simulink model "Smart_City_QCar1_self_driving_stack"  (R2024b)
settings: Solver=ode1  StartTime=0.0  StopTime=inf  FixedStep=Controller_Sample_Time  RelTol=1e-3  EnableMultiTasking=on
values from neighbouring files (symbols this model uses):
  angles_qcar1 = angles_new_qcar1(2: length (angles_new_qcar1), width (angles_new_qcar1)-5)    [Setup_QCar1and2_params.m]
  Audio_Sample_Time = 0.3    [Setup_QCar1and2_params.m]
  cal_pos = [0, 0, 0]    [Setup_QCar1and2_params.m]
  cameraStepSize = 3e-2    (= 0.03)    [Setup_QCar1and2_params.m]
  Cobra_Start = [0 0 0 0 0 0 0 0 0 0 0 0 ... (192000 elements, 192000x1)]    [QCar_Sounds.mat]
  Controller_Sample_Time = CSI_Sample_Time/10    (= 0.00166666666667)    [Setup_QCar1and2_params.m]
  CSI_Sample_Time = 1/60    (= 0.0166666666667)    [Setup_QCar1and2_params.m]
  GyroKF_P0 = eye(2)    [Setup_QCar1and2_params.m]
  GyroKF_Q = diag([0.01, 0.001])    [Setup_QCar1and2_params.m]
  GyroKF_R = 0.01    [Setup_QCar1and2_params.m]
  GyroKF_X0 = [0;0]    [Setup_QCar1and2_params.m]
  honk = [0.01708984375 0.0179443359375 0.018798828125 0.019775390625 0.0209655761719 0.0218505859375 0.0221557617188 0.0223693847656 0.022705078125 0.023681640625 0.0252075195312 0.0257263183594 ... (43568 elements, 21784x2)]    [QCar_Sounds.mat]
  ImageDisplay_Sample_Time = CSI_Sample_Time*6    (= 0.1)    [Setup_QCar1and2_params.m]
  Initialization_Time = 5    [Setup_QCar1and2_params.m]
  LiDAR_Sample_Time = CSI_Sample_Time*3    (= 0.05)    [Setup_QCar1and2_params.m]
  map_mask = [1 1 1 0 0 1 0]    [Setup_QCar1and2_params.m]
  NN_Sample_Time = RealSense_Sample_Time*1    (= 0.0333333333333)    [Setup_QCar1and2_params.m]
  path_x = [0.826 0.836 0.846 0.856 0.866 0.876 0.886 0.896 0.906 0.916 0.926 0.936 ... (740 elements, 740x1)]    [SDCS_Paths_7.mat]
  path_x2 = [-0.614 -0.604 -0.594 -0.584 -0.574 -0.564 -0.554 -0.544 -0.534 -0.524 -0.514 -0.504 ... (1090 elements, 1090x1)]    [SDCS_Paths_7.mat]
  path_x3 = [-0.614 -0.603821428571 -0.593642857143 -0.583464285714 -0.573285714286 -0.563107142857 -0.552928571429 -0.54275 -0.532571428571 -0.522392857143 -0.512214285714 -0.502035714286 ... (714 elements, 714x1)]    [SDCS_Paths_7.mat]
  path_x4 = [-0.614 -0.604 -0.594 -0.584 -0.574 -0.564 -0.554 -0.544 -0.534 -0.524 -0.514 -0.504 ... (1761 elements, 1761x1)]    [SDCS_Paths_7.mat]
  path_x5 = [1.436 1.42588571429 1.41577142857 1.40565714286 1.39554285714 1.38542857143 1.37531428571 1.3652 1.35508571429 1.34497142857 1.33485714286 1.32474285714 ... (574 elements, 574x1)]    [SDCS_Paths_7.mat]
  path_x6 = [1.436 1.42588571429 1.41577142857 1.40565714286 1.39554285714 1.38542857143 1.37531428571 1.3652 1.35508571429 1.34497142857 1.33485714286 1.32474285714 ... (1288 elements, 1288x1)]    [SDCS_Paths_7.mat]
  path_x7 = [-1.5778487585 -1.56959877056 -1.56127865467 -1.55288878259 -1.54442952915 -1.53590127231 -1.52730439309 -1.51863927561 -1.50990630701 -1.50110587746 -1.49223838016 -1.4833042113 ... (2260 elements, 2260x1)]    [SDCS_Paths_7.mat]
  path_y = [-1.0887 -1.0887 -1.0887 -1.0887 -1.0887 -1.0887 -1.0887 -1.0887 -1.0887 -1.0887 -1.0887 -1.0887 ... (740 elements, 740x1)]    [SDCS_Paths_7.mat]
  path_y2 = [-1.0887 -1.0887 -1.0887 -1.0887 -1.0887 -1.0887 -1.0887 -1.0887 -1.0887 -1.0887 -1.0887 -1.0887 ... (1090 elements, 1090x1)]    [SDCS_Paths_7.mat]
  path_y3 = [-1.0887 -1.0887 -1.0887 -1.0887 -1.0887 -1.0887 -1.0887 -1.0887 -1.0887 -1.0887 -1.0887 -1.0887 ... (714 elements, 714x1)]    [SDCS_Paths_7.mat]
  path_y4 = [-1.0887 -1.0887 -1.0887 -1.0887 -1.0887 -1.0887 -1.0887 -1.0887 -1.0887 -1.0887 -1.0887 -1.0887 ... (1761 elements, 1761x1)]    [SDCS_Paths_7.mat]
  path_y5 = [-0.8157 -0.8157 -0.8157 -0.8157 -0.8157 -0.8157 -0.8157 -0.8157 -0.8157 -0.8157 -0.8157 -0.8157 ... (574 elements, 574x1)]    [SDCS_Paths_7.mat]
  path_y6 = [-0.8157 -0.8157 -0.8157 -0.8157 -0.8157 -0.8157 -0.8157 -0.8157 -0.8157 -0.8157 -0.8157 -0.8157 ... (1288 elements, 1288x1)]    [SDCS_Paths_7.mat]
  path_y7 = [-0.614490295955 -0.61974988896 -0.624981792226 -0.630185771997 -0.635361595765 -0.640509032279 -0.645627851559 -0.6507178249 -0.655778724888 -0.660810325409 -0.665812401655 -0.670784730139 ... (2260 elements, 2260x1)]    [SDCS_Paths_7.mat]
  put_me_down = [0 0 0 0 0 0 0 0 0 0 0 0 ... (335870 elements, 167935x2)]    [QCar_Sounds.mat]
  qcar1_lidar_to_map_rotation = pi/2    (= 1.57079632679)    [Setup_QCar1and2_params.m]
  QCarEKF_L = 0.24    [Setup_QCar1and2_params.m]
  QCarEKF_P0 = eye(3)    [Setup_QCar1and2_params.m]
  QCarEKF_Q = diag([0.00001, 0.00001, 0.00001])    [Setup_QCar1and2_params.m]
  QCarEKF_R_combined = diag([0.1, 0.1, 0.01])    [Setup_QCar1and2_params.m]
  QCarEKF_R_heading = diag(0.1)    [Setup_QCar1and2_params.m]
  QcarKF_X0 = [0; 0; 0]    [Setup_QCar1and2_params.m]
  range_qcar1 = distance_new_qcar1(2: length (distance_new_qcar1), width (distance_new_qcar1)-5)    [Setup_QCar1and2_params.m]
  RealSense_Sample_Time = CSI_Sample_Time*2    (= 0.0333333333333)    [Setup_QCar1and2_params.m]
undefined symbols (not defined in the file or in its folder): DiscIntNeverNeededParam, gcbh, HIL, Joystick_Sample_Time, JPEG, Point, qc_get_step_size, video_display_show
libraries: quarc_library x63, simulink_extras x12, simulink x8
(part 1 of 5)
settings Model: SimulationMode=external  ExtModeTrigDuration=10000  Creator=PKaram  LastModifiedBy=user
settings SolverCC: AlgebraicLoopSolver=TrustRegion  PositivePriorityOrder=on  AutoInsertRateTranBlk=on
settings DataIOCC: ReturnWorkspaceOutputs=off
settings DebuggingCC: ParameterPrecisionLossMsg=none  UnconnectedInputMsg=warning  UnconnectedOutputMsg=warning  UnconnectedLineMsg=warning  ArithmeticOperatorsInVariantConditions=warning
settings HardwareCC: ProdBitPerLong=64  ProdLargestAtomicFloat=None  ProdEndianess=Unspecified  ProdHWDeviceType=Generic->64-bit Embedded Processor (LP64)
settings ModelReferenceCC: EnableRefExpFcnMdlSchedulingChecks=on
settings SFSimCC: SimUseLocalCustomCode=off  CustomCodeUndefinedFunction=UseInterfaceOnly
settings RTWCC: Description=QUARC Linux Nvidia Target (QCar) Using Toolchain  SystemTargetFile=quarc_linux_nvidia.tlc  TemplateMakefile=quarc_linux_nvidia_tmf  RTWUseLocalCustomCode=off  Toolchain=QUARC linux_nvidia | gmake (64-bit Windows)  BuildConfiguration=Faster Runs  GPUComputeCapability=3.5
settings CodeAppCC: StateflowObjectComments=on
settings STFCustomTargetCC: TargetLangStandard=C99 (ISO)  ConcurrentExecutionCompliant=on  GRTInterface=on  UseToolchainInfoCompliant=on  SystemTargetFile=quarc_linux_nvidia.tlc
settings GRTTargetCC: ParMdlRefBuildCompliant=off  CompOptLevelCompliant=off  CombineOutputUpdateFcns=off  MatFileLogging=off  CPPClassGenCompliant=off  GRTInterface=on  ExtMode=on  ExtModeMexFile=quarc_comm  ExtModeMexArgs='-w -d /tmp -uri %u', 'tcpip://192.168.2.12:17001'
settings ConfigComp: CovMetricSettings=dswe

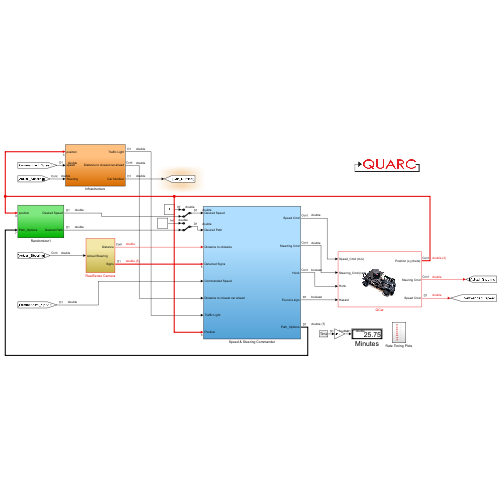
[thumbnail: Simulink's stored preview of the top-level diagram]
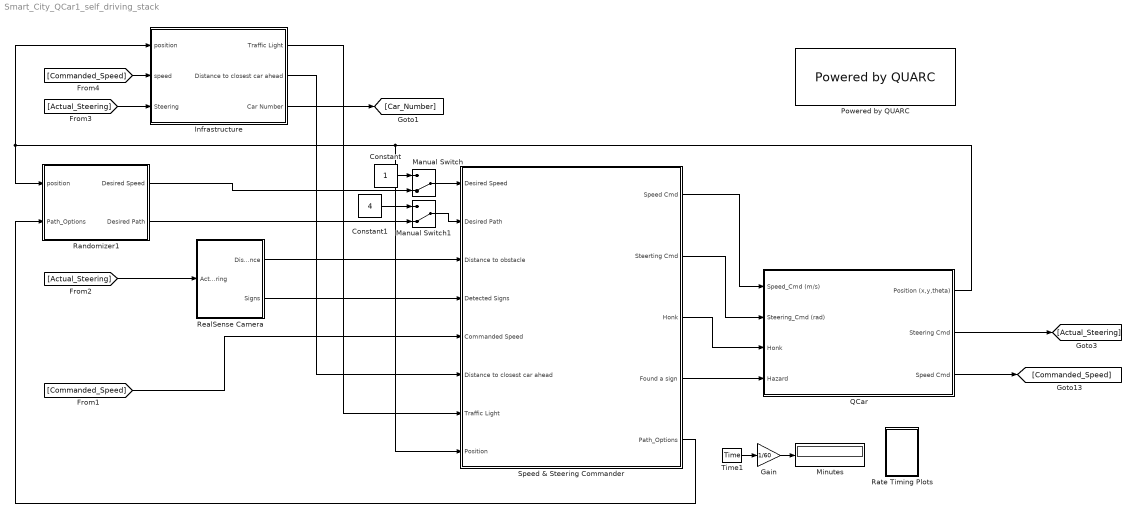
== system Smart_City_QCar1_self_driving_stack ==
  Constant : Constant
  Constant1 : Constant  Value=4
  Gain : Gain  Gain=1/60
  Infrastructure : Subsystem
  Manual Switch : ManualSwitch  CurrentSetting=0
  Manual Switch1 : ManualSwitch  CurrentSetting=0
  Minutes : Display
  Powered by QUARC : quarc_library/Logos/Powered by QUARC
  QCar : Subsystem
      mask Display: image('QCar.png'); % Use "Edit Image" on toolstrip to change.
  Randomizer1 : Subsystem
  Rate Timing Plots : Subsystem
  RealSense Camera : Subsystem
  Speed & Steering Commander : Subsystem
  Time1 : quarc_library/Sources/Time/Time  time_source=Wall clock  sample_time=qc_get_step_size
  wires:
  QCar/2(Steering Cmd) -> [Actual_Steering]
  QCar/3(Speed Cmd) -> [Commanded_Speed]
  Time1/1 -> Gain/1
  Gain/1 -> Minutes/1
  Infrastructure/1(Traffic Light) -> Speed & Steering Commander/7(Traffic Light)
  Infrastructure/2(Distance to closest car ahead) -> Speed & Steering Commander/6(Distance to closest car ahead)
  Infrastructure/3(Car Number) -> [Car_Number]
  [Actual_Steering] -> RealSense Camera/1(Actual Steering)
  [Commanded_Speed] -> Infrastructure/2("speed ")
  QCar/1(Position (x,y,theta)) -> Speed & Steering Commander/8(Position), Randomizer1/1(position), Infrastructure/1(position)
  [Actual_Steering] -> Infrastructure/3(Steering)
  [Commanded_Speed] -> Speed & Steering Commander/5(Commanded Speed)
  RealSense Camera/2(Signs) -> Speed & Steering Commander/4(Detected Signs)
  RealSense Camera/1(Distance) -> Speed & Steering Commander/3(Distance to obstacle)
  Speed & Steering Commander/4(Found a sign) -> QCar/4(Hazard)
  Speed & Steering Commander/1(Speed Cmd) -> QCar/1(Speed_Cmd (m/s))
  Speed & Steering Commander/2(Steerting Cmd) -> QCar/2(Steering_Cmd (rad))
  Speed & Steering Commander/3(Honk) -> QCar/3(Honk)
  Speed & Steering Commander/5(Path_Options) -> Randomizer1/2(Path_Options)
  Manual Switch/1 -> Speed & Steering Commander/1(Desired Speed)
  Randomizer1/1(Desired Speed) -> Manual Switch/2
  Constant/1 -> Manual Switch/1
  Randomizer1/2(Desired Path) -> Manual Switch1/2
  Constant1/1 -> Manual Switch1/1
  Manual Switch1/1 -> Speed & Steering Commander/2(Desired Path)

== system Smart_City_QCar1_self_driving_stack/Infrastructure ==
  note: Send Position and Heading to Ground Station
  note: Find:
      | 1 - Traffic light states (bool)
      | 2 - Distance to closes car for adaptive cruise control
      | 3 - Car number
  note: Get Data
  note: Make sure to change the port for each car:
      | 1: 1111
      | 2: 2222
      | 3: 3333
      | 4: 4444
      | 5: 5555
  position : Inport
  "speed " : Inport  Port=2
  Steering : Inport  Port=3
  Add : Sum
  Constant1 : Constant  Value=10
  Constant2 : Constant
  Constant4 : Constant
  Constant6 : Constant  Value=10
  Constant7 : Constant
  Demux : Demux  Outputs=[10 1 1]
  Display : Display
  Display1 : Display
  Display2 : Display
      settings: Decimation=100
  Find Closest Car : Subsystem
  Gain1 : Gain  Gain=.11537*1
  Mux : Mux  Inputs=2
  Mux3 : Mux  Inputs=2
  Saturation : Saturate  UpperLimit=1  LowerLimit=0
  Saturation1 : Saturate  UpperLimit=5  LowerLimit=1
  Second-Order Low-Pass Filter : quarc_library/Continuous/Second-Order Low-Pass Filter  params_source=External (input ports)  input_width=1  input_zeta=1  input_init=0
  Second-Order Low-Pass Filter1 : quarc_library/Continuous/Second-Order Low-Pass Filter  params_source=External (input ports)  input_width=1  input_zeta=1  input_init=0
  Selector : Selector  InputPortWidth=3  IndexOptions=Index vector (dialog)  Indices=1:2  OutputSizes=1
  Selector1 : Selector  InputPortWidth=3  IndexOptions=Index vector (dialog)  Indices=3  OutputSizes=1
  Stream Server : quarc_library/Communications/Basic/Stream Server  uri_source=Specify via dialog (do not evaluate)  uri=tcpip://remotehost:1111?nagle='off'  send_buffer_size=1460  receive_buffer_size=1460  byte_order=little endian (Intel - LSB first)  optimization=Minimum latency  send_options=Send most recent data  receive_options=Receive most recent data  default_value=10* ones (1,12)  sample_time=qc_get_step_size  active=off  implementation=Use blocking I/O in a separate thread  send_fifo_size=1  receive_fifo_size=1  send_priority=0  receive_priority=0  send_dimensions=off  receive_dimensions=off  max_dimensions=-1  data_type=Inherited via back propagation  type_expr=BusObject
      settings: AttributesFormatString="\"tcpip://remotehost:1111?nagle='off'\""
  Sum1 : Sum  Inputs=+-
  Trigonometric Function : Trigonometry  Operator=cos
  Trigonometric Function1 : Trigonometry
  Traffic Light : Outport
  Distance to closest car ahead : Outport  Port=2
  Car Number : Outport  Port=3
  wires:
  Constant7/1 -> Second-Order Low-Pass Filter/3
  Constant4/1 -> Stream Server/2
  Stream Server/1 -> Display2/1
  Constant6/1 -> Second-Order Low-Pass Filter/2
  position/1 -> Selector1/1, Selector/1
  Selector/1 -> [xy]
  Selector1/1 -> [mod_heading]
  Second-Order Low-Pass Filter/1 -> Display/1, Distance to closest car ahead/1
  Constant1/1 -> Second-Order Low-Pass Filter1/2
  "speed "/1 -> Second-Order Low-Pass Filter1/1, Second-Order Low-Pass Filter1/4
  Stream Server/4 -> Demux/1, Display1/1
  [xy] -> Find Closest Car/2(car_position)
  Constant2/1 -> Second-Order Low-Pass Filter1/3
  Second-Order Low-Pass Filter1/1 -> Find Closest Car/1("speed ")
  Find Closest Car/1(distance) -> Second-Order Low-Pass Filter/1, Second-Order Low-Pass Filter/4
  Add/1 -> Find Closest Car/3(car_heading)
  [mod_heading] -> Add/1
  Steering/1 -> Add/2
  Demux/1 -> Find Closest Car/4(other_car_position)
  Demux/2 -> Saturation/1
  Saturation/1 -> Traffic Light/1
  Mux/1 -> Stream Server/1
  Sum1/1 -> Mux/1
  [mod_heading] -> Mux/2
  Demux/3 -> Saturation1/1
  Saturation1/1 -> Car Number/1, Find Closest Car/5(car_index)
  [mod_heading] -> Trigonometric Function1/1, Trigonometric Function/1
  Mux3/1 -> Gain1/1
  Trigonometric Function1/1 -> Mux3/2
  [xy] -> Sum1/1
  Gain1/1 -> Sum1/2
  Trigonometric Function/1 -> Mux3/1

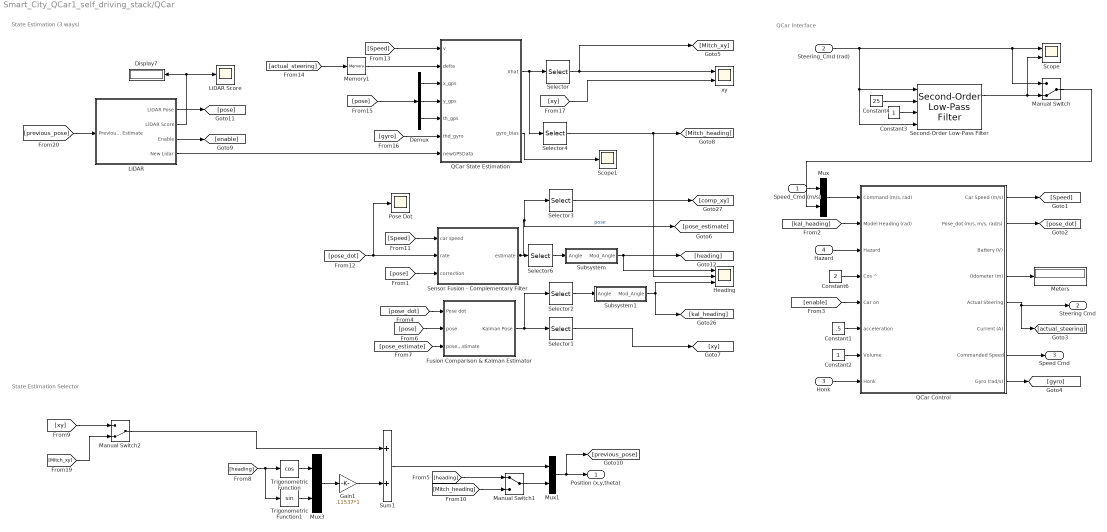
== system Smart_City_QCar1_self_driving_stack/QCar ==
  note: QCar Interface
  note: State Estimation (3 ways)
  note: State Estimation Selector
  Speed_Cmd (m/s) : Inport
  Steering_Cmd (rad) : Inport  Port=2
  Honk : Inport  Port=3
  Hazard : Inport  Port=4
  Constant1 : Constant  Value=.5
  Constant2 : Constant
  Constant3 : Constant
  Constant4 : Constant  Value=25
  Constant6 : Constant  Value=2
  Demux : Demux  Outputs=3
  Display7 : Display
  Fusion Comparison & Kalman Estimator : Subsystem
  Gain1 : Gain  Gain=.11537*1
  Heading : Scope  NumInputPorts=3
  LiDAR : Subsystem
  LiDAR Score : Scope
  Manual Switch : ManualSwitch  CurrentSetting=0
  Manual Switch1 : ManualSwitch
  Manual Switch2 : ManualSwitch  CurrentSetting=0
  Memory1 : Memory
  Meters : Display
  Mux : Mux  Inputs=2
  Mux1 : Mux  Inputs=2
  Mux3 : Mux  Inputs=2
  Pose Dot : Scope
  QCar Control : Subsystem
  QCar State Estimation : Subsystem
  Scope : Scope  NumInputPorts=2
  Scope1 : Scope
  Second-Order Low-Pass Filter : quarc_library/Continuous/Second-Order Low-Pass Filter  params_source=External (input ports)  input_width=1  input_zeta=1  input_init=0
  Selector : Selector  InputPortWidth=3  IndexOptions=Index vector (dialog)  Indices=1:2  OutputSizes=1
  Selector1 : Selector  InputPortWidth=3  IndexOptions=Index vector (dialog)  Indices=1:2  OutputSizes=1
  Selector2 : Selector  InputPortWidth=3  IndexOptions=Index vector (dialog)  Indices=3  OutputSizes=1
  Selector3 : Selector  InputPortWidth=3  IndexOptions=Index vector (dialog)  Indices=1:2  OutputSizes=1
  Selector4 : Selector  InputPortWidth=3  IndexOptions=Index vector (dialog)  Indices=3  OutputSizes=1
  Selector6 : Selector  InputPortWidth=3  IndexOptions=Index vector (dialog)  Indices=3  OutputSizes=1
  Sensor Fusion - Complementary Filter : Subsystem
  Subsystem : Subsystem
  Subsystem1 : Subsystem
  Sum1 : Sum
  Trigonometric Function : Trigonometry  Operator=cos
  Trigonometric Function1 : Trigonometry
  "xy " : Scope  NumInputPorts=2
  Position (x,y,theta) : Outport
  Steering Cmd : Outport  Port=2
  Speed Cmd : Outport  Port=3
  wires:
  Mux/1 -> QCar Control/1("Command (m/s, rad)")
  Speed_Cmd (m/s)/1 -> Mux/1
  LiDAR/2("LiDAR Score ") -> LiDAR Score/1, Display7/1
  LiDAR/1(LiDAR Pose) -> [pose]
  LiDAR/3(Enable) -> [enable]
  [pose] -> Fusion Comparison & Kalman Estimator/2(pose)
  Selector3/1 -> [comp_xy]
  [Speed] -> Sensor Fusion - Complementary Filter/1(car speed)
  Sensor Fusion - Complementary Filter/1(estimate) -> Selector3/1, [pose_estimate], Selector6/1  "pose"
  [pose_dot] -> Pose Dot/1, Sensor Fusion - Complementary Filter/2(rate)
  Selector6/1 -> Subsystem/1(Angle)
  Fusion Comparison & Kalman Estimator/1(Kalman Pose) -> Selector2/1, Selector1/1
  [pose] -> Sensor Fusion - Complementary Filter/3(correction)
  Subsystem/1(Mod_Angle) -> Heading/1, [heading]
  [pose_estimate] -> Fusion Comparison & Kalman Estimator/3(pose estimate)
  Selector2/1 -> Subsystem1/1(Angle)
  [pose_dot] -> Fusion Comparison & Kalman Estimator/1(Pose dot)
  QCar Control/1(Car Speed (m/s)) -> [Speed]
  QCar Control/2("Pose_dot (m/s, m/s, rad/s)") -> [pose_dot]
  QCar Control/5(Actual Steering) -> [actual_steering], Steering Cmd/1
  QCar Control/7(Commanded Speed) -> Speed Cmd/1
  Selector1/1 -> [xy]
  [kal_heading] -> QCar Control/2(Model Heading (rad))
  Subsystem1/1(Mod_Angle) -> Heading/3, [kal_heading]
  Constant6/1 -> QCar Control/4(Cos ^)
  Constant1/1 -> QCar Control/6(acceleration)
  [enable] -> QCar Control/5(Car on)
  Constant2/1 -> QCar Control/7(Volume)
  Honk/1 -> QCar Control/8(Honk)
  Mux1/1 -> [previous_pose], Position (x,y,theta)/1
  QCar Control/4(Odometer (m)) -> Meters/1
  Hazard/1 -> QCar Control/3(Hazard)
  Gain1/1 -> Sum1/2
  Trigonometric Function/1 -> Mux3/1
  Mux3/1 -> Gain1/1
  Trigonometric Function1/1 -> Mux3/2
  [heading] -> Trigonometric Function1/1, Trigonometric Function/1
  Sum1/1 -> Mux1/1
  Manual Switch/1 -> Mux/2
  Second-Order Low-Pass Filter/1 -> Scope/2, Manual Switch/2
  Steering_Cmd (rad)/1 -> Manual Switch/1, Scope/1, Second-Order Low-Pass Filter/1, Second-Order Low-Pass Filter/4
  Constant3/1 -> Second-Order Low-Pass Filter/3
  Constant4/1 -> Second-Order Low-Pass Filter/2
  Manual Switch1/1 -> Mux1/2
  [heading] -> Manual Switch1/1
  [Mitch_heading] -> Manual Switch1/2
  [Speed] -> QCar State Estimation/1(v)
  Demux/1 -> QCar State Estimation/3(x_gps)
  Demux/2 -> QCar State Estimation/4(y_gps)
  Demux/3 -> QCar State Estimation/5(th_gps)
  [pose] -> Demux/1
  QCar Control/8(Gyro (rad/s)) -> [gyro]
  [gyro] -> QCar State Estimation/6(thd_gyro)
  LiDAR/4(New Lidar) -> QCar State Estimation/7(newGPSData)
  QCar State Estimation/1(Xhat) -> Selector4/1, Selector/1
  [xy] -> "xy "/2
  Selector4/1 -> Heading/2, [Mitch_heading]
  QCar State Estimation/2(gyro_bias) -> Scope1/1
  Selector/1 -> [Mitch_xy], "xy "/1
  Manual Switch2/1 -> Sum1/1
  [xy] -> Manual Switch2/1
  [Mitch_xy] -> Manual Switch2/2
  [actual_steering] -> Memory1/1
  Memory1/1 -> QCar State Estimation/2(delta)
  [previous_pose] -> LiDAR/1(Previous Estimate)

== system Smart_City_QCar1_self_driving_stack/Randomizer1 ==
  note: Tunable Params
  position : Inport
  Path_Options : Inport  Port=2
  Base Speed : Constant  Value=.35
  Compare To Constant : simulink/Logic and Bit Operations/Compare To Constant  relop=<  const=0  OutDataTypeStr=boolean
  Compare To Constant1 : simulink/Logic and Bit Operations/Compare To Constant  relop=>  const=-0.75  OutDataTypeStr=boolean
  Compare To Constant2 : simulink/Logic and Bit Operations/Compare To Constant  relop=<  const=-0.9  OutDataTypeStr=boolean
  Display : Display
  Display1 : Display
  Logical Operator : Logic  AllPortsSameDT=off  OutDataTypeStr=boolean
  Logical Operator1 : Logic  AllPortsSameDT=off  OutDataTypeStr=boolean
  MATLAB Function : MATLAB Function  TreatAsAtomicUnit=on
  Memory1 : Memory  InitialCondition=2  InheritSampleTime=on  LinearizeMemory=on  LinearizeAsDelay=on
  Memory2 : Memory  InitialCondition=1  InheritSampleTime=on  LinearizeMemory=on  LinearizeAsDelay=on
  Subsystem1 : Subsystem
  Terminator : Terminator
  Time b/w Path Changes : Constant  Value=3
  X : Selector  InputPortWidth=3  IndexOptions=Index vector (dialog)  Indices=[1]  OutputSizes=1
  Y : Selector  InputPortWidth=3  IndexOptions=Index vector (dialog)  Indices=[2]  OutputSizes=1
  multiply : Product  Inputs=**
  select which which path set to use : Subsystem  TreatAsAtomicUnit=on
  Desired Speed : Outport
  Desired Path : Outport  Port=2
  wires:
  Memory1/1 -> MATLAB Function/1(Previous_Path)
  Memory2/1 -> MATLAB Function/2(Previous_Speed)
  Time b/w Path Changes/1 -> Subsystem1/1(Random Period)
  Subsystem1/1(RisingEdgeTrigger) -> MATLAB Function/5(randomize)
  Base Speed/1 -> MATLAB Function/4(Speed_Cmd_Base)
  MATLAB Function/2(Desired_Speed) -> Desired Speed/1, Memory2/1, Display1/1
  MATLAB Function/1(Desired_Path) -> Memory1/1, Desired Path/1, Display/1
  MATLAB Function/3(Accel_Limit) -> Terminator/1
  X/1 -> Compare To Constant1/1, Compare To Constant/1
  Logical Operator/1 -> Logical Operator1/1
  Compare To Constant1/1 -> Logical Operator/2
  position/1 -> X/1, Y/1
  Logical Operator1/1 -> select which which path set to use/Trigger
  select which which path set to use/1(map mask) -> multiply/1
  Y/1 -> Compare To Constant2/1
  Compare To Constant/1 -> Logical Operator/1
  Compare To Constant2/1 -> Logical Operator1/2
  Path_Options/1 -> multiply/2
  multiply/1 -> MATLAB Function/3(Path_Options)

== system Smart_City_QCar1_self_driving_stack/Rate Timing Plots ==
  Audio : Scope
  CSI : Scope
  Control : Scope
  Image Displays : Scope
  Joystick : Scope  Commented=on
  LCD : Scope
  LiDAR : Scope
  NN Rate : Scope
  RealSense : Scope
  monitorTiming : Subsystem
  monitorTiming1 : Subsystem
  monitorTiming2 : Subsystem
  monitorTiming3 : Subsystem
  monitorTiming4 : Subsystem  Commented=on
  monitorTiming5 : Subsystem
  monitorTiming6 : Subsystem
  monitorTiming7 : Subsystem
  monitorTiming8 : Subsystem
  wires:
  monitorTiming/1(Timing (s)) -> CSI/1
  monitorTiming1/1(Timing (s)) -> Control/1
  monitorTiming3/1(Timing (s)) -> Image Displays/1
  monitorTiming4/1(Timing (s)) -> Joystick/1
  monitorTiming2/1(Timing (s)) -> RealSense/1
  monitorTiming5/1(Timing (s)) -> LiDAR/1
  monitorTiming6/1(Timing (s)) -> NN Rate/1
  monitorTiming7/1(Timing (s)) -> LCD/1
  monitorTiming8/1(Timing (s)) -> Audio/1

== system Smart_City_QCar1_self_driving_stack/RealSense Camera ==
  note: Capture Realsense and get object distance
  Actual Steering : Inport
  Constant8 : Constant  Value=50
  Constant9 : Constant
  NN Classification : Scope
  Newer Depth : Subsystem  LoadFcn=set_param(gcbh, 'UserData', gcb);  StartFcn=video_display_show([gcb, '/Video Display'], 'add', gcb);  mask(Video Compressed Display){algorithm=JPEG, quality=50, sample_time=-1, use_hardware=on}
      mask prompts: algorithm "Compression algorithm:"; quality "Compression quality (0-100):"; sample_time "Sample time (seconds):"; use_hardware "Use hardware acceleration for video display"
      mask help: Displays a video stream on the host, using compression to minimize bandwidth.
      mask init:
      | qc_set_display('Video\nCompressed\nDisplay');
      settings: UndoDeleteFcn=set_param(gcbh, 'UserData', gcb);  OpenFcn=video_display_show([gcb, '/Video Display'], 'show', gcb);  PreDeleteFcn=video_display_show([gcb, '/Video Display'], 'delete');
      settings: CopyFcn=|
      | set_param(gcbh, 'UserData', gcb);
      | set_param(gcbh, 'LinkStatus', 'none');
      settings: NameChangeFcn=|
      | video_display_show([get_param(gcbh, 'UserData'), '/Video Display'], 'rename', [gcb, '/Video Display']);
      | video_display_show([gcb, '/Video Display'], 'add', gcb);
      | set_param(gcbh, 'UserData', gcb);
      mask Help: web(qc_get_block_help_path(gcb));
      mask TypeOptions algorithm: Image Compress/algorithm
      mask TypeOptions quality: Image Compress/quality
      mask TypeOptions sample_time: Video Display/sample_time
      mask TypeOptions use_hardware: Video Display/use_hardware
      mask Display:
      | patch([0.98591 0.98591 0.62618 0.59072 0.56147   0.536   0.536  0.5441 0.56912 0.59207 0.60881 0.62276 0.63527 0.64364  0.6485  0.6485 0.64706 0.64499 0.63662 0.62411 0.61232 0.59837 0.58307 0.56147   0.536   0.536  0.5441  0.5747 0.60953 0.63662 0.67001  0.7034 0.72851 0.75425 0.77927 0.80294 0.82454 0.84119 0.85865 0.87395 0.88574 0.89339  0.8969 0.89969 0.89969 0.89267  0.8816 0.87044 0.85649  0.8384 0.81824 0.80294 0.78764 0.77513 0.76676 0.75776 0.76397 0.77513 0.79178 0.80987 0.82796 0.84326 0.86207 0.98528],[0.18689 0.05522 0.05522 0.05171 0.05171    0.05 0.18338 0.18338 0.19148 0.20435 0.22298 0.24863 0.28589 0.33125 0.38138 0.55139 0.59801 0.63761 0.68189 0.72149 0.74939 0.76694 0.77855 0.79367 0.79952 0.92768 0.92768 0.92768 0.92417 0.92066 0.91364  0.9032 0.89384 0.88106 0.86594 0.85073 0.82634 0.80537 0.77855 0.74363 0.70403 0.65858 0.61079 0.59099 0.41513 0.37202 0.31847 0.29048 0.25556 0.23342  0.2102 0.19382 0.18221 0.17285 0.16943 0.16124  0.1589 0.16241 0.16709 0.17168  0.1787 0.18221 0.18689 0.18689],[0.9,0.90,0.91])
      | patch([0.536 0.52601 0.46823 0.44528 0.41603 0.39101 0.35555 0.33116 0.31451 0.29291  0.2804 0.26717 0.25322 0.23999 0.22406 0.20732 0.19337 0.17528 0.15935 0.14396 0.13217 0.11759 0.10922 0.10085 0.09671 0.09392 0.09041 0.08906 0.08906 0.09464  0.0995 0.10778 0.11894 0.13145 0.14675 0.16349 0.17672 0.19409 0.20732 0.22406 0.23999 0.26159 0.27833 0.29849 0.31793 0.33602 0.35411 0.37085 0.39245 0.41603   0.536   0.536 0.53159 0.46409   0.446 0.42026 0.39587 0.37571 0.36113 0.34925 0.34088 0.33809 0.33809 0.34088 0.34583 0.35627 0.36392 0.38129 0.39587 0.41117 0.42719 0.44672  0.4676 0.48353 0.48353 0.52394   0.536],[0.05 0.04829 0.04712 0.04712 0.04829 0.05063 0.05405 0.05873 0.06107 0.06692 0.07043 0.07619 0.08087 0.08672 0.09482 0.10652 0.11696 0.13325  0.1508 0.17168 0.19499 0.22415 0.25439 0.28472 0.31379 0.35456 0.38489 0.41513 0.58055 0.63878 0.68774 0.72149 0.75641 0.78089 0.80537 0.82859 0.84029 0.85658 0.86594 0.87404  0.8834 0.89267 0.90086 0.90788 0.91247 0.91832 0.92066   0.923 0.92651 0.92768 0.92768 0.79952 0.79952 0.79952 0.79718 0.78899 0.77153 0.75056 0.72149 0.68072 0.62249  0.5549 0.41396 0.37085 0.33242 0.28121 0.25205 0.22181 0.20552 0.19499 0.18572 0.18221 0.17753 0.17636 0.17753  0.1787  0.1787],[0.9,0.90,0.91])
      | disp('Video\nCompressed\nDisplay');
  RGB : Subsystem  LoadFcn=set_param(gcbh, 'UserData', gcb);  StartFcn=video_display_show([gcb, '/Video Display'], 'add', gcb);  mask(Video Compressed Display){algorithm=JPEG, quality=50, sample_time=-1, use_hardware=on}
      mask prompts: algorithm "Compression algorithm:"; quality "Compression quality (0-100):"; sample_time "Sample time (seconds):"; use_hardware "Use hardware acceleration for video display"
      mask help: Displays a video stream on the host, using compression to minimize bandwidth.
      mask init:
      | qc_set_display('Video\nCompressed\nDisplay');
      settings: UndoDeleteFcn=set_param(gcbh, 'UserData', gcb);  OpenFcn=video_display_show([gcb, '/Video Display'], 'show', gcb);  PreDeleteFcn=video_display_show([gcb, '/Video Display'], 'delete');
      settings: CopyFcn=|
      | set_param(gcbh, 'UserData', gcb);
      | set_param(gcbh, 'LinkStatus', 'none');
      settings: NameChangeFcn=|
      | video_display_show([get_param(gcbh, 'UserData'), '/Video Display'], 'rename', [gcb, '/Video Display']);
      | video_display_show([gcb, '/Video Display'], 'add', gcb);
      | set_param(gcbh, 'UserData', gcb);
      mask Help: web(qc_get_block_help_path(gcb));
      mask TypeOptions algorithm: Image Compress/algorithm
      mask TypeOptions quality: Image Compress/quality
      mask TypeOptions sample_time: Video Display/sample_time
      mask TypeOptions use_hardware: Video Display/use_hardware
      mask Display:
      | patch([0.98591 0.98591 0.62618 0.59072 0.56147   0.536   0.536  0.5441 0.56912 0.59207 0.60881 0.62276 0.63527 0.64364  0.6485  0.6485 0.64706 0.64499 0.63662 0.62411 0.61232 0.59837 0.58307 0.56147   0.536   0.536  0.5441  0.5747 0.60953 0.63662 0.67001  0.7034 0.72851 0.75425 0.77927 0.80294 0.82454 0.84119 0.85865 0.87395 0.88574 0.89339  0.8969 0.89969 0.89969 0.89267  0.8816 0.87044 0.85649  0.8384 0.81824 0.80294 0.78764 0.77513 0.76676 0.75776 0.76397 0.77513 0.79178 0.80987 0.82796 0.84326 0.86207 0.98528],[0.18689 0.05522 0.05522 0.05171 0.05171    0.05 0.18338 0.18338 0.19148 0.20435 0.22298 0.24863 0.28589 0.33125 0.38138 0.55139 0.59801 0.63761 0.68189 0.72149 0.74939 0.76694 0.77855 0.79367 0.79952 0.92768 0.92768 0.92768 0.92417 0.92066 0.91364  0.9032 0.89384 0.88106 0.86594 0.85073 0.82634 0.80537 0.77855 0.74363 0.70403 0.65858 0.61079 0.59099 0.41513 0.37202 0.31847 0.29048 0.25556 0.23342  0.2102 0.19382 0.18221 0.17285 0.16943 0.16124  0.1589 0.16241 0.16709 0.17168  0.1787 0.18221 0.18689 0.18689],[0.9,0.90,0.91])
      | patch([0.536 0.52601 0.46823 0.44528 0.41603 0.39101 0.35555 0.33116 0.31451 0.29291  0.2804 0.26717 0.25322 0.23999 0.22406 0.20732 0.19337 0.17528 0.15935 0.14396 0.13217 0.11759 0.10922 0.10085 0.09671 0.09392 0.09041 0.08906 0.08906 0.09464  0.0995 0.10778 0.11894 0.13145 0.14675 0.16349 0.17672 0.19409 0.20732 0.22406 0.23999 0.26159 0.27833 0.29849 0.31793 0.33602 0.35411 0.37085 0.39245 0.41603   0.536   0.536 0.53159 0.46409   0.446 0.42026 0.39587 0.37571 0.36113 0.34925 0.34088 0.33809 0.33809 0.34088 0.34583 0.35627 0.36392 0.38129 0.39587 0.41117 0.42719 0.44672  0.4676 0.48353 0.48353 0.52394   0.536],[0.05 0.04829 0.04712 0.04712 0.04829 0.05063 0.05405 0.05873 0.06107 0.06692 0.07043 0.07619 0.08087 0.08672 0.09482 0.10652 0.11696 0.13325  0.1508 0.17168 0.19499 0.22415 0.25439 0.28472 0.31379 0.35456 0.38489 0.41513 0.58055 0.63878 0.68774 0.72149 0.75641 0.78089 0.80537 0.82859 0.84029 0.85658 0.86594 0.87404  0.8834 0.89267 0.90086 0.90788 0.91247 0.91832 0.92066   0.923 0.92651 0.92768 0.92768 0.79952 0.79952 0.79952 0.79718 0.78899 0.77153 0.75056 0.72149 0.68072 0.62249  0.5549 0.41396 0.37085 0.33242 0.28121 0.25205 0.22181 0.20552 0.19499 0.18572 0.18221 0.17753 0.17636 0.17753  0.1787  0.1787],[0.9,0.90,0.91])
      | disp('Video\nCompressed\nDisplay');
  Rate Transition : RateTransition
  Rate Transition2 : RateTransition
  Rate Transition4 : RateTransition
  RealSense Capture : Subsystem
  Second-Order Low-Pass Filter2 : quarc_library/Continuous/Second-Order Low-Pass Filter  params_source=External (input ports)  input_width=1  input_zeta=1  input_init=0
  Terminator : Terminator
  Transfer Fcn : TransferFcn  Numerator=[10]  Denominator=[1 10]
  obstacleDetection Markham March 22 : Subsystem
  to 16Hz4 : RateTransition  OutPortSampleTime=ImageDisplay_Sample_Time
  Distance : Outport
  Signs : Outport  Port=2
  wires:
  Transfer Fcn/1 -> Rate Transition4/1
  Actual Steering/1 -> Transfer Fcn/1
  Constant9/1 -> Second-Order Low-Pass Filter2/3
  obstacleDetection Markham March 22/2(distance (m)) -> Rate Transition2/1
  Rate Transition2/1 -> Second-Order Low-Pass Filter2/4, Second-Order Low-Pass Filter2/1
  to 16Hz4/1 -> Newer Depth/1(In1)
  obstacleDetection Markham March 22/1(imageDepthForDisplay) -> to 16Hz4/1
  Second-Order Low-Pass Filter2/2 -> Terminator/1
  RealSense Capture/1(New) -> obstacleDetection Markham March 22/Enable
  RealSense Capture/2(Depth) -> obstacleDetection Markham March 22/1(imageDepth)
  Rate Transition4/1 -> obstacleDetection Markham March 22/2(steering (rad))
  Constant8/1 -> Second-Order Low-Pass Filter2/2
  Second-Order Low-Pass Filter2/1 -> Distance/1
  RealSense Capture/3(RGB Image) -> RGB/1(In1)
  RealSense Capture/4(Sign Probabilities) -> Rate Transition/1, NN Classification/1
  Rate Transition/1 -> Signs/1

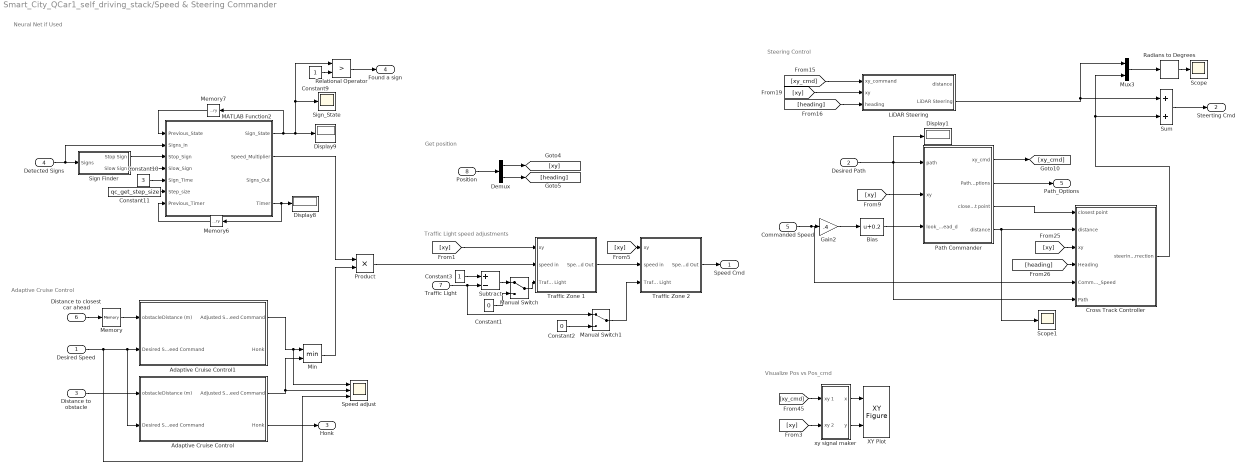
== system Smart_City_QCar1_self_driving_stack/Speed & Steering Commander ==
  note: Get position
  note: Steering Control
  note: Visualize Pos vs Pos_cmd
  note: Traffic Light speed adjustments
  note: Adaptive Cruise Control
  note: Neural Net if Used
  Desired Speed : Inport
  Desired Path : Inport  Port=2
  Distance to obstacle : Inport  Port=3
  Detected Signs : Inport  Port=4
  Commanded Speed : Inport  Port=5
  Distance to closest car ahead : Inport  Port=6
  Traffic Light : Inport  Port=7
  Position : Inport  Port=8
  Adaptive Cruise Control : Subsystem
  Adaptive Cruise Control1 : Subsystem
  Bias : Bias  Bias=0.2  SaturateOnIntegerOverflow=off
  Constant1 : Constant  Value=0
  Constant10 : Constant  Value=3
  Constant11 : Constant  Value=qc_get_step_size
  Constant2 : Constant  Value=0
  Constant3 : Constant
  Constant9 : Constant
  Cross Track Controller : Subsystem
  Demux : Demux  Outputs=2
  Display1 : Display
  Display8 : Display
  Display9 : Display
  Gain2 : Gain  Gain=.4
  LiDAR Steering : Subsystem
  MATLAB Function2 : MATLAB Function  TreatAsAtomicUnit=on
  Manual Switch : ManualSwitch
  Manual Switch1 : ManualSwitch
  Memory : Memory  InheritSampleTime=on  LinearizeMemory=on  LinearizeAsDelay=on
  Memory6 : Memory  InheritSampleTime=on  LinearizeMemory=on  LinearizeAsDelay=on
  Memory7 : Memory  InitialCondition=1  InheritSampleTime=on  LinearizeMemory=on  LinearizeAsDelay=on
  Min : MinMax  Inputs=2
  Mux3 : Mux  Inputs=2
  Path Commander : Subsystem
  Product : Product
  Radians to Degrees : simulink_extras/Transformations/Radians to Degrees
  Relational Operator : RelationalOperator  Operator=>  OutDataTypeStr=boolean  RndMeth=Simplest  InputSameDT=off
  Scope : Scope
  Scope1 : Scope
  Sign Finder : Subsystem
  Sign_State : Scope
  Speed adjust : Scope  NumInputPorts=3
  Subtract : Sum  Inputs=+-
  Sum : Sum
  Traffic Zone 1 : Subsystem
  Traffic Zone 2 : Subsystem
  XY Plot : quarc_library/Sinks/Figures/XY Figure  figure_mode=Use figure window  figure_tag=figure1  axes_tag=axes1  plot_mode=Time-based  minimum_x=-2.5  maximum_x=2.5  minimum_y=-2  maximum_y=5  buffer_size=100  update_rate=1  initial_position="-958  549  958  474"  initial_visibility=off  sample_time=-1
      settings: SourceProductName=QUARC Targets
  xy signal maker : Subsystem
  Speed Cmd : Outport
  Steerting Cmd : Outport  Port=2
  Honk : Outport  Port=3
  Found a sign : Outport  Port=4
  Path_Options : Outport  Port=5
  wires:
  [heading] -> LiDAR Steering/3(heading)
  Bias/1 -> Path Commander/3(look_ahead_d)
  Relational Operator/1 -> Found a sign/1
  [xy] -> Cross Track Controller/3(xy)
  Gain2/1 -> Bias/1
  [heading] -> Cross Track Controller/4(Heading)
  Memory6/1 -> MATLAB Function2/7(Previous_Timer)
  Constant9/1 -> Relational Operator/2
  Constant11/1 -> MATLAB Function2/6(Step_size)
  MATLAB Function2/1(Sign_State) -> Display9/1, Relational Operator/1, Sign_State/1, Memory7/1
  Commanded Speed/1 -> Cross Track Controller/5(Commanded_Speed), Gain2/1
  [xy] -> Path Commander/2(xy)
  Mux3/1 -> Radians to Degrees/1
  MATLAB Function2/4(Timer) -> Display8/1, Memory6/1
  Constant10/1 -> MATLAB Function2/5(Sign_Time)
  [xy_cmd] -> LiDAR Steering/1(xy_command)
  Desired Path/1 -> Cross Track Controller/6(Path), Path Commander/1(path), Display1/1
  Memory7/1 -> MATLAB Function2/1(Previous_State)
  LiDAR Steering/2(LiDAR Steering) -> Mux3/1, Sum/1
  [xy] -> LiDAR Steering/2(xy)
  Path Commander/3(closest point) -> Cross Track Controller/1(closest point)
  Sign Finder/1(Stop Sign) -> MATLAB Function2/3(Stop_Sign)
  Path Commander/1(xy_cmd) -> [xy_cmd]
  Cross Track Controller/1(steering correction) -> Mux3/2, Sum/2
  Radians to Degrees/1 -> Scope/1
  Path Commander/4(distance) -> Scope1/1, Cross Track Controller/2(distance)
  Sign Finder/2(Slow Sign) -> MATLAB Function2/4(Slow_Sign)
  Distance to obstacle/1 -> Adaptive Cruise Control/1(obstacleDistance (m))
  Desired Speed/1 -> Speed adjust/3, Adaptive Cruise Control1/2(Desired Speed Command), Adaptive Cruise Control/2(Desired Speed Command)
  Demux/2 -> [heading]
  Position/1 -> Demux/1
  Demux/1 -> [xy]
  Detected Signs/1 -> MATLAB Function2/2(Signs_In), Sign Finder/1(Signs)
  Sum/1 -> Steerting Cmd/1
  MATLAB Function2/2(Speed_Multiplier) -> Product/1
  Adaptive Cruise Control/2(Honk) -> Honk/1
  xy signal maker/2(y) -> XY Plot/2
  [xy_cmd] -> xy signal maker/1(xy 1)
  [xy] -> xy signal maker/2(xy 2)
  xy signal maker/1(x) -> XY Plot/1
  Traffic Zone 1/1(Speed Out) -> Traffic Zone 2/2(speed in)
  Constant3/1 -> Subtract/1
  [xy] -> Traffic Zone 2/1(xy)
  [xy] -> Traffic Zone 1/1(xy)
  Traffic Zone 2/1(Speed Out) -> Speed Cmd/1
  Product/1 -> Traffic Zone 1/2(speed in)
  Distance to closest car ahead/1 -> Memory/1
  Min/1 -> Product/2
  Adaptive Cruise Control1/1(Adjusted Speed Command) -> Speed adjust/1, Min/1
  Adaptive Cruise Control/1(Adjusted Speed Command) -> Min/2, Speed adjust/2
  Memory/1 -> Adaptive Cruise Control1/1(obstacleDistance (m))
  Path Commander/2(Path_Options) -> Path_Options/1
  Traffic Light/1 -> Manual Switch1/1, Subtract/2
  Subtract/1 -> Manual Switch/1
  Manual Switch/1 -> Traffic Zone 1/3(Traffic Light)
  Constant1/1 -> Manual Switch/2
  Constant2/1 -> Manual Switch1/2
  Manual Switch1/1 -> Traffic Zone 2/3(Traffic Light)

== system Smart_City_QCar1_self_driving_stack/Infrastructure/Find Closest Car ==
  "speed " : Inport
  car_position : Inport  Port=2
  car_heading : Inport  Port=3
  other_car_position : Inport  Port=4
  car_index : Inport  Port=5
  Constant1 : Constant  Value=65
  Constant2 : Constant  Value=45
  Constant6 : Constant
  Constant7 : Constant
  Constant8 : Constant  Value=10
  Degrees to Radians : simulink_extras/Transformations/Degrees to Radians
  Demux : Demux  Outputs=2
  Demux1 : Demux  Outputs=2
  Display{,1..3} (4 alike) : Display
      settings: Decimation=100
  MATLAB Function : MATLAB Function  TreatAsAtomicUnit=on
  MATLAB Function1 : MATLAB Function  TreatAsAtomicUnit=on
  Radians to Degrees : simulink_extras/Transformations/Radians to Degrees
  Saturation Dynamic : simulink/Discontinuities/Saturation Dynamic  OutMin=[]  OutMax=[]  OutDataTypeStr=Inherit: Same as second input  OutDataType=fixdt(1, 16)  OutScaling=2^-10  DoSatur=off
  distance : Outport
  wires:
  Constant6/1 -> MATLAB Function/7(proximity_radius)
  Constant8/1 -> MATLAB Function/9(max_distance)
  car_index/1 -> MATLAB Function/5(car_index)
  Radians to Degrees/1 -> Display2/1
  car_heading/1 -> MATLAB Function/6(heading)
  MATLAB Function/2(distance_vector) -> Display1/1
  Degrees to Radians/1 -> MATLAB Function/8(proximity_scan_window)
  MATLAB Function/3(heading_vector) -> Radians to Degrees/1
  MATLAB Function/1(distance) -> Display/1, distance/1
  Demux/1 -> MATLAB Function/1(x_car)
  Demux/2 -> MATLAB Function/2(y_car)
  car_position/1 -> Demux/1
  other_car_position/1 -> Demux1/1
  Demux1/1 -> MATLAB Function/3(x_vector)
  Demux1/2 -> MATLAB Function/4(y_vector)
  "speed "/1 -> MATLAB Function1/1(speed)
  Constant7/1 -> MATLAB Function1/2(max_speed)
  Constant1/1 -> Saturation Dynamic/1, MATLAB Function1/4(max_window)
  Constant2/1 -> Saturation Dynamic/3, MATLAB Function1/3(min_window)
  MATLAB Function1/1(proximity_scan_window) -> Saturation Dynamic/2
  Saturation Dynamic/1 -> Display3/1, Degrees to Radians/1

== system Smart_City_QCar1_self_driving_stack/QCar/Fusion Comparison & Kalman Estimator ==
  Pose dot : Inport
  pose : Inport  Port=2
  pose estimate : Inport  Port=3
  Angle mod1 : Subsystem
  Constant : Constant  Value=3
  Data Type Conversion1 : DataTypeConversion  OutDataTypeStr=int32  RndMeth=Round  SaturateOnIntegerOverflow=off
  Data Type Conversion2 : DataTypeConversion  OutDataTypeStr=int32  RndMeth=Round  SaturateOnIntegerOverflow=off
  Heading : Scope
  Integrator : Integrator  ExternalReset=level  InitialConditionSource=external  WrappedStateUpperValue=[20 20 pi]  WrappedStateLowerValue=-[20 20 pi]
  Kalman : Selector  InputPortWidth=3  IndexOptions=Index vector (port)  Indices=[1 3]  OutputSizes=1
  LiDAR : Selector  InputPortWidth=3  IndexOptions=Index vector (port)  Indices=[1 3]  OutputSizes=1
  LiDAR1 : Selector  InputPortWidth=3  IndexOptions=Index vector (port)  Indices=[1 3]  OutputSizes=1
  Memory2 : Memory  InheritSampleTime=on  LinearizeMemory=on  LinearizeAsDelay=on
  Mux : Mux  Inputs=2
  Mux1 : Mux  Inputs=2
  Mux2 : Mux  Inputs=2
  Mux4 : Mux  Inputs=3
  RT : RateTransition  OutPortSampleTime=qc_get_step_size
  RT1 : RateTransition  OutPortSampleTime=qc_get_step_size
  RT2 : RateTransition  OutPortSampleTime=qc_get_step_size
  Radians to Degrees : simulink_extras/Transformations/Radians to Degrees
  Radians to Degrees2 : simulink_extras/Transformations/Radians to Degrees
  Radians to Degrees3 : simulink_extras/Transformations/Radians to Degrees
  Relational Operator1 : RelationalOperator  Operator=~=  OutDataTypeStr=boolean  RndMeth=Simplest  InputSameDT=off
  Scope : Scope  NumInputPorts=3
  Selector1 : Selector  InputPortWidth=3  IndexOptions=Index vector (dialog)  Indices=1:2  OutputSizes=1
  Selector2 : Selector  InputPortWidth=3  IndexOptions=Index vector (dialog)  Indices=3  OutputSizes=1
  Selector3 : Selector  InputPortWidth=3  IndexOptions=Index vector (dialog)  Indices=1:2  OutputSizes=1
  Selector4 : Selector  InputPortWidth=3  IndexOptions=Index vector (dialog)  Indices=3  OutputSizes=1
  Selector5 : Selector  InputPortWidth=3  IndexOptions=Index vector (dialog)  Indices=1:2  OutputSizes=1
  Selector6 : Selector  InputPortWidth=3  IndexOptions=Index vector (dialog)  Indices=3  OutputSizes=1
  Selector7 : Selector  InputPortWidth=3  IndexOptions=Index vector (dialog)  Indices=1  OutputSizes=1
  m_to_mm : Gain  Gain=1e3
  m_to_mm1 : Gain  Gain=1e3
  m_to_mm2 : Gain  Gain=1e3
  Kalman Pose : Outport
  wires:
  Mux2/1 -> LiDAR1/1, Scope/3
  Selector6/1 -> Radians to Degrees3/1
  m_to_mm2/1 -> Mux2/1
  Integrator/1 -> Kalman Pose/1, Selector1/1, Selector2/1  "pose"
  Selector1/1 -> m_to_mm/1
  pose estimate/1 -> Selector6/1, Selector5/1
  Selector5/1 -> m_to_mm2/1
  Selector4/1 -> Radians to Degrees2/1
  Radians to Degrees3/1 -> Mux2/2
  Mux/1 -> Scope/1, Kalman/1, Data Type Conversion2/1
  m_to_mm1/1 -> Mux1/1
  Selector2/1 -> Radians to Degrees/1
  Pose dot/1 -> Integrator/1
  m_to_mm/1 -> Mux/1
  Mux1/1 -> Data Type Conversion1/1, RT/1
  Radians to Degrees/1 -> Mux/2
  Selector3/1 -> m_to_mm1/1
  Radians to Degrees2/1 -> Mux1/2
  RT/1 -> LiDAR/1, Scope/2
  pose/1 -> Selector7/1, Selector4/1, Selector3/1, RT2/1
  RT2/1 -> Integrator/3
  RT1/1 -> Memory2/1, Relational Operator1/2
  Memory2/1 -> Relational Operator1/1
  Selector7/1 -> RT1/1
  Relational Operator1/1 -> Integrator/2
  Mux4/1 -> Angle mod1/1(Angle)
  LiDAR/1 -> Mux4/2
  Kalman/1 -> Mux4/1
  LiDAR1/1 -> Mux4/3
  Constant/1 -> LiDAR1/2, LiDAR/2, Kalman/2
  Angle mod1/1(Mod_Angle) -> Heading/1

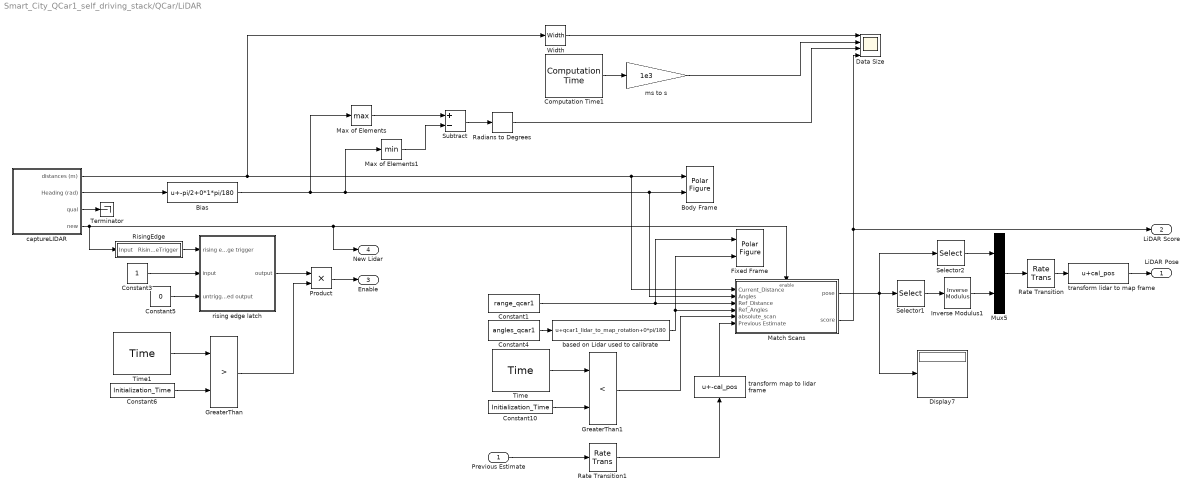
== system Smart_City_QCar1_self_driving_stack/QCar/LiDAR ==
  Previous Estimate : Inport
  Bias : Bias  Bias=-pi/2+0*1*pi/180  SaturateOnIntegerOverflow=off
  Body Frame : quarc_library/Sinks/Figures/Polar Figure  figure_mode=Use figure window  figure_tag=figure1  axes_tag=axes1  plot_mode=Frame-based  minimum_rho=0  maximum_rho=8  minimum_theta=0  maximum_theta=360  zero_location=right  direction=clockwise  buffer_size=SPR_qcar1  update_rate=1  sample_time=-1  initial_position="1.8            50         766.4           806"  initial_visibility=off  line1_style=None  line1_width=0.5  line1_color=[0 0.4470 0.7410]  marker1=Point (.)  marker1_size=1  marker1_edge_color=[0 0.447059 0.741176]  marker1_face_color=[0 0.447059 0.741176]  line2_style=Solid line (-)  line2_width=0.5  line2_color=[0.85098 0.32549 0.0980392]  marker2=None  marker2_size=6  marker2_edge_color=[0.85098 0.32549 0.0980392]  marker2_face_color=[0.85098 0.32549 0.0980392]  line3_style=Solid line (-)  line3_width=0.5  line3_color=[0.929412 0.694118 0.12549]  marker3=None  marker3_size=6  marker3_edge_color=[0.929412 0.694118 0.12549]  marker3_face_color=[0.929412 0.694118 0.12549]  line4_style=Solid line (-)  line4_width=0.5  line4_color=[0.494118 0.184314 0.556863]  marker4=None  marker4_size=6  marker4_edge_color=[0.494118 0.184314 0.556863]  marker4_face_color=[0.494118 0.184314 0.556863]  line5_style=Solid line (-)  line5_width=0.5  line5_color=[0.466667 0.67451 0.188235]  marker5=None  marker5_size=6  marker5_edge_color=[0.466667 0.67451 0.188235]  marker5_face_color=[0.466667 0.67451 0.188235]
      settings: SourceProductName=QUARC Targets
  Computation Time1 : quarc_library/Sources/Time/Computation Time  sample_time=LiDAR_Sample_Time  use_model=on  use_cpu_time=off
  Constant1 : Constant  Value=range_qcar1
  Constant10 : Constant  Value=Initialization_Time
  Constant3 : Constant
  Constant4 : Constant  Value=angles_qcar1
  Constant5 : Constant  Value=0
  Constant6 : Constant  Value=Initialization_Time
  Data Size : Scope  NumInputPorts=4
  Display7 : Display
  Fixed Frame : quarc_library/Sinks/Figures/Polar Figure  figure_mode=Use figure window  figure_tag=figure1  axes_tag=axes1  plot_mode=Frame-based  minimum_rho=0  maximum_rho=5  minimum_theta=0  maximum_theta=360  zero_location=right  direction=clockwise  buffer_size=SPR_qcar1  update_rate=1  sample_time=-1  initial_position="275 -108  958  981"  initial_visibility=off  line1_style=None  line1_width=0.5  line1_color=[0 0.4470 0.7410]  marker1=Point (.)  marker1_size=1  marker1_edge_color=[0 0.447059 0.741176]  marker1_face_color=[0 0.447059 0.741176]  line2_style=Solid line (-)  line2_width=0.5  line2_color=[0.85098 0.32549 0.0980392]  marker2=None  marker2_size=6  marker2_edge_color=[0.85098 0.32549 0.0980392]  marker2_face_color=[0.85098 0.32549 0.0980392]  line3_style=Solid line (-)  line3_width=0.5  line3_color=[0.929412 0.694118 0.12549]  marker3=None  marker3_size=6  marker3_edge_color=[0.929412 0.694118 0.12549]  marker3_face_color=[0.929412 0.694118 0.12549]  line4_style=Solid line (-)  line4_width=0.5  line4_color=[0.494118 0.184314 0.556863]  marker4=None  marker4_size=6  marker4_edge_color=[0.494118 0.184314 0.556863]  marker4_face_color=[0.494118 0.184314 0.556863]  line5_style=Solid line (-)  line5_width=0.5  line5_color=[0.466667 0.67451 0.188235]  marker5=None  marker5_size=6  marker5_edge_color=[0.466667 0.67451 0.188235]  marker5_face_color=[0.466667 0.67451 0.188235]
      settings: SourceProductName=QUARC Targets
  GreaterThan : RelationalOperator  Operator=>  OutDataTypeStr=boolean  RndMeth=Simplest  InputSameDT=off
  GreaterThan1 : RelationalOperator  Operator=<  OutDataTypeStr=boolean  RndMeth=Simplest  InputSameDT=off
  Inverse Modulus1 : quarc_library/Discontinuities/Inverse Modulus  modulus=2*pi  output_derivative=off  output_revolutions=off  max_x=Inf  min_x=-Inf
  Match Scans : Subsystem
  Max of Elements : MinMax  Function=max
  Max of Elements1 : MinMax
  Mux5 : Mux  Inputs=2
  Product : Product
  Radians to Degrees : simulink_extras/Transformations/Radians to Degrees
  Rate Transition : RateTransition
  Rate Transition1 : RateTransition
  RisingEdge : Subsystem
  Selector1 : Selector  InputPortWidth=3  IndexOptions=Index vector (dialog)  Indices=3  OutputSizes=1
  Selector2 : Selector  InputPortWidth=3  IndexOptions=Index vector (dialog)  Indices=1:2  OutputSizes=1
  Subtract : Sum  Inputs=+-
  Terminator : Terminator
  Time : quarc_library/Sources/Time/Time  time_source=Wall clock  sample_time=LiDAR_Sample_Time
  Time1 : quarc_library/Sources/Time/Time  time_source=Wall clock  sample_time=qc_get_step_size
  Width : Width
  based on Lidar used to calibrate : Bias  Bias=qcar1_lidar_to_map_rotation+0*pi/180  SaturateOnIntegerOverflow=off
  captureLIDAR : Subsystem
  ms to s : Gain  Gain=1e3
  rising edge latch : Subsystem
  transform lidar to map frame : Bias  Bias=cal_pos  SaturateOnIntegerOverflow=off
  transform map to lidar frame : Bias  Bias=-cal_pos  SaturateOnIntegerOverflow=off
  LiDAR Pose : Outport
  "LiDAR Score " : Outport  Port=2
  Enable : Outport  Port=3
  New Lidar : Outport  Port=4
  wires:
  Constant1/1 -> Fixed Frame/1, Match Scans/3(Ref_Distance)
  Width/1 -> Data Size/1
  captureLIDAR/1(distances (m)) -> Width/1, Match Scans/1(Current_Distance), Body Frame/1
  Computation Time1/1 -> ms to s/1
  Max of Elements/1 -> Subtract/1
  ms to s/1 -> Data Size/2
  Max of Elements1/1 -> Subtract/2
  Match Scans/1(pose) -> Selector2/1, Selector1/1, Display7/1
  Inverse Modulus1/1 -> Mux5/2
  Selector2/1 -> Mux5/1
  Radians to Degrees/1 -> Data Size/3
  Selector1/1 -> Inverse Modulus1/1
  Constant6/1 -> GreaterThan/2
  RisingEdge/1(RisingEdgeTrigger) -> rising edge latch/1(rising edge trigger)
  Match Scans/2(score) -> Data Size/4, "LiDAR Score "/1
  Product/1 -> Enable/1
  Constant3/1 -> rising edge latch/2(input)
  Constant5/1 -> rising edge latch/3(untriggered output)
  Constant10/1 -> GreaterThan1/2
  GreaterThan/1 -> Product/2
  Subtract/1 -> Radians to Degrees/1
  Time/1 -> GreaterThan1/1
  GreaterThan1/1 -> Match Scans/5(absolute_scan)
  Time1/1 -> GreaterThan/1
  captureLIDAR/2(Heading (rad)) -> Bias/1
  rising edge latch/1(output) -> Product/1
  Bias/1 -> Max of Elements/1, Max of Elements1/1, Body Frame/2, Match Scans/2(Angles)
  captureLIDAR/4(new) -> RisingEdge/1(Input), New Lidar/1, Match Scans/Enable
  transform lidar to map frame/1 -> LiDAR Pose/1
  Rate Transition/1 -> transform lidar to map frame/1
  Mux5/1 -> Rate Transition/1
  Rate Transition1/1 -> transform map to lidar frame/1
  transform map to lidar frame/1 -> Match Scans/6(Previous Estimate)
  Previous Estimate/1 -> Rate Transition1/1
  captureLIDAR/3(qual) -> Terminator/1
  based on Lidar used to calibrate/1 -> Match Scans/4(Ref_Angles), Fixed Frame/2
  Constant4/1 -> based on Lidar used to calibrate/1
